simulink model "Kinematic_Bicycle_Model"  (R2020a)
settings: Solver=VariableStepAuto  StartTime=0.0  StopTime=10  RelTol=1e-3
values from neighbouring files (symbols this model uses):
  delta_max = deg2rad(37.3)    [init.m]
  initial_psi = 0    [init.m]
  initial_x0 = 0    [init.m]
  initial_y0 = 0    [init.m]
  input_velocity = v_lon0    (= 5)    [init.m]
  kd = -0.0238    [init.m]
  kp = -0.0235    [init.m]
  length_front = 1.04    [init.m]
  length_rare = 1.4    [init.m]
  steering_constant = deg2rad(10)    [init.m]
  steering_input_switch = 3    [init.m]
  steering_omega = 0.25    [init.m]
  steering_rate = deg2rad(2)    [init.m]
libraries: simulink x2
settings Model: Creator=Sameed Quais  LastModifiedBy=Sameed Quais

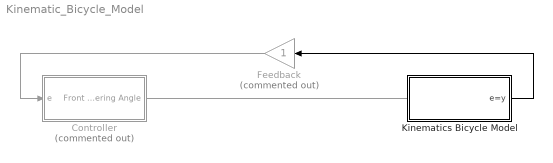
== system Kinematic_Bicycle_Model ==
  Controller : Subsystem  Commented=on
  Feedback : Gain  Commented=on
  Kinematics Bicycle Model : Subsystem
  wires:
  Controller/1("Front Wheel Steering Angle ") -> ?
  Kinematics Bicycle Model/1(e=y) -> Feedback/1
  Feedback/1 -> Controller/1(e)

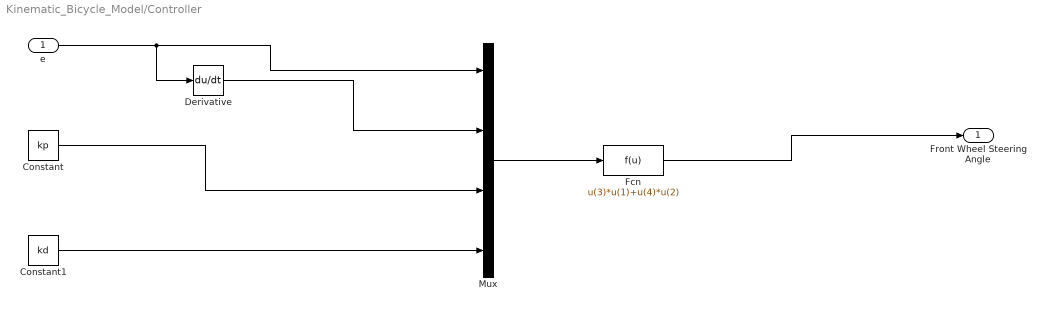
== system Kinematic_Bicycle_Model/Controller ==
  e : Inport
  Constant : Constant  Value=kp
  Constant1 : Constant  Value=kd
  Derivative : Derivative
  Fcn : Fcn  Expr=u(3)*u(1)+u(4)*u(2)
  Mux : Mux
  "Front Wheel Steering Angle " : Outport
  wires:
  e/1 -> Derivative/1, Mux/1
  Derivative/1 -> Mux/2
  Constant/1 -> Mux/3
  Constant1/1 -> Mux/4
  Mux/1 -> Fcn/1
  Fcn/1 -> "Front Wheel Steering Angle "/1

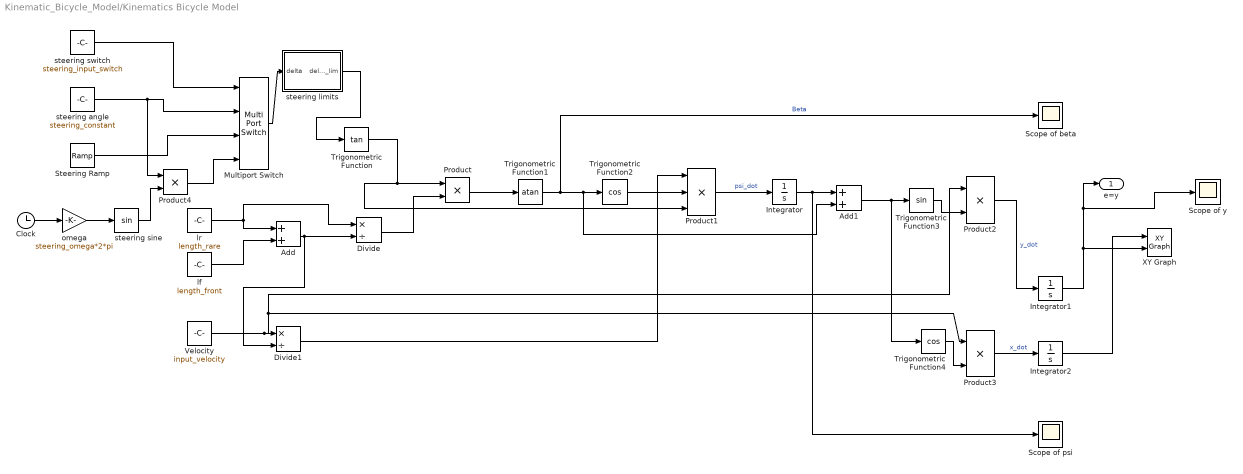
== system Kinematic_Bicycle_Model/Kinematics Bicycle Model ==
  Add : Sum
  Add1 : Sum
  Clock : Clock
  Divide : Product  Inputs=*/
  Divide1 : Product  Inputs=*/
  Integrator : Integrator  InitialCondition=initial_psi
  Integrator1 : Integrator  InitialCondition=initial_y0
  Integrator2 : Integrator  InitialCondition=initial_x0
  Multiport Switch : MultiPortSwitch
  Product{,2..4} (4 alike) : Product
  Product1 : Product  Inputs=3
  Scope of beta : Scope
  Scope of psi : Scope
  Scope of y : Scope
  Steering Ramp : simulink/Sources/Ramp  slope=steering_rate  start=0  InitialOutput=0
  Trigonometric Function : Trigonometry  Operator=tan
  Trigonometric Function1 : Trigonometry  Operator=atan
  Trigonometric Function2 : Trigonometry  Operator=cos
  Trigonometric Function3 : Trigonometry
  Trigonometric Function4 : Trigonometry  Operator=cos
  Velocity : Constant  Value=input_velocity
  XY Graph : simulink/Sinks/XY Graph  xmin=-inf  xmax=inf  ymin=-inf  ymax=inf  st=-1
  lf : Constant  Value=length_front
  lr : Constant  Value=length_rare
  omega : Gain  Gain=steering_omega*2*pi
  steering limits : Subsystem
  steering angle : Constant  Value=steering_constant
  steering sine : Trigonometry
  steering switch : Constant  Value=steering_input_switch
  e=y : Outport
  wires:
  lr/1 -> Divide/1, Add/1
  lf/1 -> Add/2
  Trigonometric Function/1 -> Product1/3, Product/1
  Add/1 -> Divide1/2, Divide/2
  Divide/1 -> Product/2
  Product/1 -> Trigonometric Function1/1
  Trigonometric Function1/1 -> Scope of beta/1, Add1/2, Trigonometric Function2/1  "Beta"
  Trigonometric Function2/1 -> Product1/2
  Velocity/1 -> Product2/1, Product3/1, Divide1/1
  Divide1/1 -> Product1/1
  Product1/1 -> Integrator/1  "psi_dot"
  Integrator/1 -> Scope of psi/1, Add1/1
  Add1/1 -> Trigonometric Function4/1, Trigonometric Function3/1
  Trigonometric Function3/1 -> Product2/2
  Product2/1 -> Integrator1/1  "y_dot"
  Trigonometric Function4/1 -> Product3/2
  Product3/1 -> Integrator2/1  "x_dot"
  Integrator1/1 -> Scope of y/1, e=y/1, XY Graph/2
  Integrator2/1 -> XY Graph/1
  steering switch/1 -> Multiport Switch/1
  steering angle/1 -> Product4/1, Multiport Switch/2
  Steering Ramp/1 -> Multiport Switch/3
  omega/1 -> steering sine/1
  Clock/1 -> omega/1
  steering sine/1 -> Product4/2
  Product4/1 -> Multiport Switch/4
  Multiport Switch/1 -> steering limits/1(delta)
  steering limits/1(delta_lim) -> Trigonometric Function/1

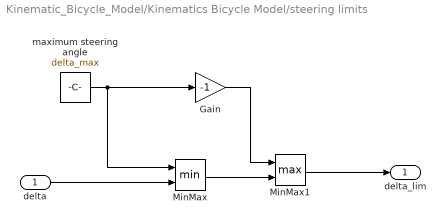
== system Kinematic_Bicycle_Model/Kinematics Bicycle Model/steering limits ==
  delta : Inport
  Gain : Gain  Gain=-1
  MinMax : MinMax  Inputs=2
  MinMax1 : MinMax  Function=max  Inputs=2
  maximum steering angle : Constant  Value=delta_max
  delta_lim : Outport  VectorParamsAs1DForOutWhenUnconnected=off
  wires:
  MinMax1/1 -> delta_lim/1
  delta/1 -> MinMax/2
  maximum steering angle/1 -> Gain/1, MinMax/1
  MinMax/1 -> MinMax1/2
  Gain/1 -> MinMax1/1
